simulink model "SSN_39busRT_Ctrl_4WT_19B"  (R2021a)
settings: Solver=ode3  StartTime=0.0  StopTime=10  FixedStep=Ts  MaxStep=1/60  RelTol=1e-2  AbsTol=1e-1
PreLoadFcn:
  | Ts=2.50e-6; ssn_ieee39_params; load('Pwf.mat');
InitFcn:
  | Ts=2.50e-6; ssn_ieee39_params; load('Pwf.mat');
values from neighbouring files (symbols this model uses):
  f = 50    [ssn_ieee39_params_ctrl.m]
  fNom = f    (= 60)    [ssn_ieee39_params_ctrl.m]
  ILR = 5.02    [ssn_ieee39_params_ctrl.m]
  IQMIN = 0.1    [ssn_ieee39_params_ctrl.m]
  ISCLIM = 1    [ssn_ieee39_params_ctrl.m]
  ITFpu = 1.10    (= 1.1)    [ssn_ieee39_params_ctrl.m]
  K = 1    [ssn_ieee39_params_ctrl.m]
  K1 = 1    [ssn_ieee39_params_ctrl.m]
  K2 = 2    [ssn_ieee39_params_ctrl.m]
  KCL = 1.04    [ssn_ieee39_params_ctrl.m]
  KFB = 0    [ssn_ieee39_params_ctrl.m]
  KFF = 1    [ssn_ieee39_params_ctrl.m]
  KFIX = 1    [ssn_ieee39_params_ctrl.m]
  KG = 1    [ssn_ieee39_params_ctrl.m]
  KIA = 59.91    [ssn_ieee39_params_ctrl.m]
  KIOEX = 0.0303    [ssn_ieee39_params_ctrl.m]
  KIUEX = 0.0303    [ssn_ieee39_params_ctrl.m]
  KIUOEX = 1    [ssn_ieee39_params_ctrl.m]
  KIUUEX = 1    [ssn_ieee39_params_ctrl.m]
  KLR = 22.47    [ssn_ieee39_params_ctrl.m]
  KM = 1    [ssn_ieee39_params_ctrl.m]
  KOEL = 0.24    [ssn_ieee39_params_ctrl.m]
  Kp = 1    [ssn_ieee39_params_ctrl.m]
  KPA = 30    [ssn_ieee39_params_ctrl.m]
  KPOEL = 1    [ssn_ieee39_params_ctrl.m]
  KPOEX = 0    [ssn_ieee39_params_ctrl.m]
  KPUEX = 0    [ssn_ieee39_params_ctrl.m]
  KSCALE = 0.319    [ssn_ieee39_params_ctrl.m]
  KUF = 0    [ssn_ieee39_params_ctrl.m]
  KUI = 0.001    [ssn_ieee39_params_ctrl.m]
  KUL = 0.24    [ssn_ieee39_params_ctrl.m]
  s = 10    [ssn_ieee39_params_ctrl.m]
  TA = 0.01    [ssn_ieee39_params_ctrl.m]
  Tadj = 0    [ssn_ieee39_params_ctrl.m]
  taps = [1 1 1.07 1.07 1.009 1.025 1 1.025 1.025 1.025]*1    [ssn_ieee39_params_ctrl.m]
  TF = 0.02    [ssn_ieee39_params_ctrl.m]
  TG = 0.024    [ssn_ieee39_params_ctrl.m]
  TINV = 0    [ssn_ieee39_params_ctrl.m]
  TIT = 0.1    [ssn_ieee39_params_ctrl.m]
  TL_10_11_len = 14    [ssn_ieee39_params_ctrl.m]
  TL_10_13_len = 14    [ssn_ieee39_params_ctrl.m]
  TL_13_14_len = 32    [ssn_ieee39_params_ctrl.m]
  TL_14_15_len = 70    [ssn_ieee39_params_ctrl.m]
  TL_15_16_len = 31.5    [ssn_ieee39_params_ctrl.m]
  TL_16_17_len = 26    [ssn_ieee39_params_ctrl.m]
  TL_16_19_len = 61    [ssn_ieee39_params_ctrl.m]
  TL_16_21_len = 46    [ssn_ieee39_params_ctrl.m]
  TL_16_24_len = 15    [ssn_ieee39_params_ctrl.m]
  TL_17_18_len = 26    [ssn_ieee39_params_ctrl.m]
  TL_17_27_len = 59    [ssn_ieee39_params_ctrl.m]
  TL_1_2_len = 134    [ssn_ieee39_params_ctrl.m]
  TL_1_39_len = 105    [ssn_ieee39_params_ctrl.m]
  TL_21_22_len = 47    [ssn_ieee39_params_ctrl.m]
  TL_22_23_len = 33    [ssn_ieee39_params_ctrl.m]
  TL_24_23_len = 88    [ssn_ieee39_params_ctrl.m]
  TL_25_26_len = 101    [ssn_ieee39_params_ctrl.m]
  TL_26_27_len = 46.5    [ssn_ieee39_params_ctrl.m]
  TL_26_28_len = 151    [ssn_ieee39_params_ctrl.m]
  TL_26_29_len = 200    [ssn_ieee39_params_ctrl.m]
  TL_28_29_len = 48    [ssn_ieee39_params_ctrl.m]
  TL_2_25_len = 28    [ssn_ieee39_params_ctrl.m]
  TL_2_2_len = 49    [ssn_ieee39_params_ctrl.m]
  TL_3_18_len = 42    [ssn_ieee39_params_ctrl.m]
  TL_3_4_len = 53    [ssn_ieee39_params_ctrl.m]
  TL_4_14_len = 33    [ssn_ieee39_params_ctrl.m]
  TL_4_5_len = 32.5    [ssn_ieee39_params_ctrl.m]
  TL_5_6_len = 14    [ssn_ieee39_params_ctrl.m]
  TL_5_8_len = 32    [ssn_ieee39_params_ctrl.m]
  TL_6_11_len = 26.5    [ssn_ieee39_params_ctrl.m]
  TL_6_7_len = 25.5    [ssn_ieee39_params_ctrl.m]
  TL_7_8_len = 15    [ssn_ieee39_params_ctrl.m]
  TL_8_9_len = 93    [ssn_ieee39_params_ctrl.m]
  TL_9_39_len = 136    [ssn_ieee39_params_ctrl.m]
  TOEL = 5.00    (= 5)    [ssn_ieee39_params_ctrl.m]
  TQREF = 0    [ssn_ieee39_params_ctrl.m]
  TQSCL = 0.012    [ssn_ieee39_params_ctrl.m]
  Ts_PMU = 1/1000    (= 0.001)    [ssn_ieee39_params_ctrl.m]
  TU1 = 0    [ssn_ieee39_params_ctrl.m]
  TU2 = 0    [ssn_ieee39_params_ctrl.m]
  TU3 = 0    [ssn_ieee39_params_ctrl.m]
  TU4 = 0    [ssn_ieee39_params_ctrl.m]
  TUL = 0    [ssn_ieee39_params_ctrl.m]
  TUP = 0.050    (= 0.05)    [ssn_ieee39_params_ctrl.m]
  TUQ = .005    (= 0.005)    [ssn_ieee39_params_ctrl.m]
  TUV = 0.2    [ssn_ieee39_params_ctrl.m]
  VAAMAX = VAMAX    (= 7.05)    [ssn_ieee39_params_ctrl.m]
  VAMAX = 7.05    [ssn_ieee39_params_ctrl.m]
  VAMIN = -6.11    [ssn_ieee39_params_ctrl.m]
  VBMAX = 999    [ssn_ieee39_params_ctrl.m]
  VF = 0    [ssn_ieee39_params_ctrl.m]
  VFB = 0    [ssn_ieee39_params_ctrl.m]
  VMMAX = 7.05    [ssn_ieee39_params_ctrl.m]
  VMMIN = -6.11    [ssn_ieee39_params_ctrl.m]
  VOELmax1 = 0.2353    [ssn_ieee39_params_ctrl.m]
  VOELmax2 = 0.0    (= 0)    [ssn_ieee39_params_ctrl.m]
  VOELmin1 = -0.24    [ssn_ieee39_params_ctrl.m]
  VOELmin2 = -1.0    (= -1)    [ssn_ieee39_params_ctrl.m]
  VRMAX = 7.05    [ssn_ieee39_params_ctrl.m]
  VRMIN = -6.11    [ssn_ieee39_params_ctrl.m]
  VSCLmax = 0.20    (= 0.2)    [ssn_ieee39_params_ctrl.m]
  VSCLmin = -0.10    (= -0.1)    [ssn_ieee39_params_ctrl.m]
  VUELmax1 = 1    [ssn_ieee39_params_ctrl.m]
  VUELmax2 = 1    [ssn_ieee39_params_ctrl.m]
  VUELmin1 = -1    [ssn_ieee39_params_ctrl.m]
  VUELmin2 = -1    [ssn_ieee39_params_ctrl.m]
  VUImax = 1    [ssn_ieee39_params_ctrl.m]
  VUImin = -1    [ssn_ieee39_params_ctrl.m]
undefined symbols (not defined in the file or in its folder): another_event_name, D1, Delta, DiscIntNeverNeededParam, find_system, MOV_segment9, my_event_name, powergui, Pw1, Pw2, Pw3, Pw4, vNomHV
libraries: powerlib_extras x162, spsThreePhaseVIMeasurementLib x55, spsCurrentMeasurementLib x52, simulink_extras x44, slpidlib x40, op_dpl_lib x36, spsST2AModel x20, spsThreePhaseParallelRLCLoadLib x20, spsThreePhaseTransformerTwoWindingsLib x17, spsControlledVoltageSourceLib x16, spsVoltageMeasurementLib x12, spsSynchronousMachinepuStandardLib x10
(part 6 of 19)

== system SSN_39busRT_Ctrl_4WT_19B/powergui/EquivalentModel16/Yout ==
  v,i : Inport
  Demux : Demux  Outputs=[1 1 1 1 1 1 1 1 1 1 1 1]
  tag scope: T56_4730_4741406695273=global, T56_4731_4743248439477=global, T56_4732_4745660404880=global, T72_6441_8594295325773=global, T72_6442_8596923134147=global, T72_6443_8599741842799=global, T80_6661_10245256504684=global, T80_6662_10243102637747=global, T80_6662_10245911720449=global, T80_6663_10243756033361=global, T80_6663_10246790665215=global, T80_6664_10244633157975=global
  wires:
  v,i/1 -> Demux/1
  Demux/1 -> [T72_6441_8594295325773]
  Demux/2 -> [T72_6442_8596923134147]
  Demux/3 -> [T72_6443_8599741842799]
  Demux/4 -> [T56_4730_4741406695273]
  Demux/5 -> [T56_4732_4745660404880]
  Demux/6 -> [T56_4731_4743248439477]
  Demux/7 -> [T80_6661_10245256504684]
  Demux/8 -> [T80_6662_10245911720449]
  Demux/9 -> [T80_6663_10246790665215]
  Demux/10 -> [T80_6662_10243102637747]
  Demux/11 -> [T80_6663_10243756033361]
  Demux/12 -> [T80_6664_10244633157975]

== system SSN_39busRT_Ctrl_4WT_19B/powergui/EquivalentModel17/Sources ==
  Mux : Mux  Inputs=[2 1 1 1 1 1 1 1 1 1]
  u : Outport  VectorParamsAs1DForOutWhenUnconnected=off
  wires:
  Mux/1 -> u/1
  [T65_5743_7340394662837] -> Mux/1
  [T76_6245_8362305392589] -> Mux/2
  [T76_6246_8363477414484] -> Mux/3
  [T76_6247_8364872173221] -> Mux/4
  [T75_6196_8146580275268] -> Mux/5
  [T75_6197_8147667563989] -> Mux/6
  [T75_6198_8148974225777] -> Mux/7
  [T75_6196_8148676870836] -> Mux/8
  [T75_6197_8149763564695] -> Mux/9
  [T75_6198_8151069631622] -> Mux/10

== system SSN_39busRT_Ctrl_4WT_19B/powergui/EquivalentModel17/Yout ==
  v,i : Inport
  Demux : Demux  Outputs=[2 1 1 1 1 1 1 1 1 1 1 1 1 1 1 1 1 1 1 1 1 1 1 1 1 1 1 1]
  tag scope: T55_4653_4627484077960=global, T55_4654_4629568952949=global, T55_4655_4631788251212=global, T56_4727_4745233583373=global, T56_4728_4743871655841=global, T56_4728_4747080717351=global, T56_4729_4742591329737=global, T56_4729_4745716943000=global, T56_4729_4749498425805=global, T56_4730_4741392605062=global, T56_4730_4744434770078=global, T56_4730_4748132683584=global, T56_4731_4739957074542=global, T56_4731_4743234198584=global, T56_4731_4746848542792=global, T56_4732_4741796921701=global, T56_4732_4745646003429=global, T56_4733_4744206865714=global, T65_5738_7276287426115=global, T78_6554_9761341477516=global, T78_6554_9763216670330=global, T78_6555_9761848914346=global, T78_6555_9763723549584=global, T78_6556_9762573376817=global, T78_6556_9764447454479=global, T79_6603_10014042814288=global, T79_6604_10014630189419=global, T79_6605_10015437941512=global
  wires:
  v,i/1 -> Demux/1
  Demux/1 -> [T65_5738_7276287426115]
  Demux/2 -> [T56_4727_4745233583373]
  Demux/3 -> [T56_4729_4749498425805]
  Demux/4 -> [T56_4728_4747080717351]
  Demux/5 -> [T56_4728_4743871655841]
  Demux/6 -> [T56_4730_4748132683584]
  Demux/7 -> [T56_4729_4745716943000]
  Demux/8 -> [T56_4729_4742591329737]
  Demux/9 -> [T56_4731_4746848542792]
  Demux/10 -> [T56_4730_4744434770078]
  Demux/11 -> [T56_4730_4741392605062]
  Demux/12 -> [T56_4732_4745646003429]
  Demux/13 -> [T56_4731_4743234198584]
  Demux/14 -> [T56_4731_4739957074542]
  Demux/15 -> [T56_4733_4744206865714]
  Demux/16 -> [T56_4732_4741796921701]
  Demux/17 -> [T79_6603_10014042814288]
  Demux/18 -> [T79_6604_10014630189419]
  Demux/19 -> [T79_6605_10015437941512]
  Demux/20 -> [T78_6554_9761341477516]
  Demux/21 -> [T78_6555_9761848914346]
  Demux/22 -> [T78_6556_9762573376817]
  Demux/23 -> [T78_6554_9763216670330]
  Demux/24 -> [T78_6555_9763723549584]
  Demux/25 -> [T78_6556_9764447454479]
  Demux/26 -> [T55_4653_4627484077960]
  Demux/27 -> [T55_4654_4629568952949]
  Demux/28 -> [T55_4655_4631788251212]

== system SSN_39busRT_Ctrl_4WT_19B/powergui/EquivalentModel18/Sources ==
  Mux : Mux  Inputs=[1 1 1 1 1 1]
  u : Outport  VectorParamsAs1DForOutWhenUnconnected=off
  wires:
  Mux/1 -> u/1
  [T76_6246_8359372382981] -> Mux/1
  [T76_6247_8360543323472] -> Mux/2
  [T76_6248_8361937000805] -> Mux/3
  [T76_6249_8355395478954] -> Mux/4
  [T76_6250_8356560405551] -> Mux/5
  [T76_6251_8357948068989] -> Mux/6

== system SSN_39busRT_Ctrl_4WT_19B/powergui/EquivalentModel18/Yout ==
  v,i : Inport
  Demux : Demux  Outputs=[1 1 1 1 1 1 1 1 1]
  tag scope: T56_4732_4739239959997=global, T56_4733_4741077859883=global, T56_4734_4743485728987=global, T79_6604_10010967878637=global, T79_6605_10011554239309=global, T79_6606_10012360976943=global, T79_6607_10005727568997=global, T79_6608_10006308288062=global, T79_6609_10007109384090=global
  wires:
  v,i/1 -> Demux/1
  Demux/1 -> [T56_4732_4739239959997]
  Demux/2 -> [T56_4734_4743485728987]
  Demux/3 -> [T56_4733_4741077859883]
  Demux/4 -> [T79_6604_10010967878637]
  Demux/5 -> [T79_6605_10011554239309]
  Demux/6 -> [T79_6606_10012360976943]
  Demux/7 -> [T79_6607_10005727568997]
  Demux/8 -> [T79_6608_10006308288062]
  Demux/9 -> [T79_6609_10007109384090]

== system SSN_39busRT_Ctrl_4WT_19B/powergui/EquivalentModel19/Sources ==
  Mux : Mux  Inputs=[1 1 1 1 1 1 1 1 1 1 1 1 1 1 1]
  u : Outport  VectorParamsAs1DForOutWhenUnconnected=off
  wires:
  Mux/1 -> u/1
  [T76_6248_8355999055039] -> Mux/1
  [T76_6249_8357166447881] -> Mux/2
  [T76_6250_8358556577565] -> Mux/3
  [T76_6250_8352783092665] -> Mux/4
  [T76_6251_8353946937858] -> Mux/5
  [T76_6252_8355333519893] -> Mux/6
  [T76_6252_8350236052370] -> Mux/7
  [T76_6253_8351396140089] -> Mux/8
  [T76_6254_8352778964651] -> Mux/9
  [T76_6245_8360654367305] -> Mux/10
  [T76_6246_8361827648147] -> Mux/11
  [T76_6247_8363223665832] -> Mux/12
  [T76_6248_8355359545726] -> Mux/13
  [T76_6249_8356527190358] -> Mux/14
  [T76_6250_8357917571832] -> Mux/15

== system SSN_39busRT_Ctrl_4WT_19B/powergui/EquivalentModel19/Yout ==
  v,i : Inport
  Demux : Demux  Outputs=[1 1 1 1 1 1 1 1 1 1 1 1 1 1 1 1 1 1]
  tag scope: T56_4733_4738286039607=global, T56_4734_4740122092675=global, T56_4735_4742527993909=global, T79_6603_10012751864210=global, T79_6604_10013340420354=global, T79_6605_10014149353460=global, T79_6606_10006333101250=global, T79_6606_10006888715093=global, T79_6607_10006916370091=global, T79_6607_10007471747731=global, T79_6608_10002961019338=global, T79_6608_10007720015894=global, T79_6608_10008275157332=global, T79_6609_10003540723944=global, T79_6610_10004340805511=global, T79_6610_9999627275735=global, T79_6611_10000203455472=global, T79_6612_10001000012171=global
  wires:
  v,i/1 -> Demux/1
  Demux/1 -> [T56_4733_4738286039607]
  Demux/2 -> [T56_4735_4742527993909]
  Demux/3 -> [T56_4734_4740122092675]
  Demux/4 -> [T79_6606_10006888715093]
  Demux/5 -> [T79_6607_10007471747731]
  Demux/6 -> [T79_6608_10008275157332]
  Demux/7 -> [T79_6608_10002961019338]
  Demux/8 -> [T79_6609_10003540723944]
  Demux/9 -> [T79_6610_10004340805511]
  Demux/10 -> [T79_6610_9999627275735]
  Demux/11 -> [T79_6611_10000203455472]
  Demux/12 -> [T79_6612_10001000012171]
  Demux/13 -> [T79_6603_10012751864210]
  Demux/14 -> [T79_6604_10013340420354]
  Demux/15 -> [T79_6605_10014149353460]
  Demux/16 -> [T79_6606_10006333101250]
  Demux/17 -> [T79_6607_10006916370091]
  Demux/18 -> [T79_6608_10007720015894]

== system SSN_39busRT_Ctrl_4WT_19B/powergui/EquivalentModel2/Sources ==
  Mux : Mux  Inputs=[1 1]
  u : Outport  VectorParamsAs1DForOutWhenUnconnected=off
  wires:
  Mux/1 -> u/1
  [T160_13858_40016383632279] -> Mux/1
  [T161_13907_39894470939587] -> Mux/2

== system SSN_39busRT_Ctrl_4WT_19B/powergui/EquivalentModel2/Yout ==
  v,i : Inport
  Demux : Demux  Outputs=[1 1 1]
  tag scope: T150_12991_36851941643877=global, T167_14636_46271938604014=global, T168_14685_46271433640443=global
  wires:
  v,i/1 -> Demux/1
  Demux/1 -> [T167_14636_46271938604014]
  Demux/2 -> [T168_14685_46271433640443]
  Demux/3 -> [T150_12991_36851941643877]

== system SSN_39busRT_Ctrl_4WT_19B/powergui/EquivalentModel20/Sources ==
  Mux : Mux  Inputs=[1 1 1 1 1 1]
  u : Outport  VectorParamsAs1DForOutWhenUnconnected=off
  wires:
  Mux/1 -> u/1
  [T76_6252_8349724495860] -> Mux/1
  [T76_6253_8350884793404] -> Mux/2
  [T76_6254_8352267827789] -> Mux/3
  [T75_6200_8142991377200] -> Mux/4
  [T75_6201_8144069994674] -> Mux/5
  [T75_6202_8145367985214] -> Mux/6

== system SSN_39busRT_Ctrl_4WT_19B/powergui/EquivalentModel20/Yout ==
  v,i : Inport
  Demux : Demux  Outputs=[1 1 1 1 1 1 1 1 1]
  tag scope: T56_4735_4736623003114=global, T56_4736_4738455362545=global, T56_4737_4740857328039=global, T78_6558_9755856196192=global, T78_6559_9756355505283=global, T78_6560_9757071840015=global, T79_6610_9999184791373=global, T79_6611_9999761167945=global, T79_6612_10000557921480=global
  wires:
  v,i/1 -> Demux/1
  Demux/1 -> [T56_4735_4736623003114]
  Demux/2 -> [T56_4737_4740857328039]
  Demux/3 -> [T56_4736_4738455362545]
  Demux/4 -> [T79_6610_9999184791373]
  Demux/5 -> [T79_6611_9999761167945]
  Demux/6 -> [T79_6612_10000557921480]
  Demux/7 -> [T78_6558_9755856196192]
  Demux/8 -> [T78_6559_9756355505283]
  Demux/9 -> [T78_6560_9757071840015]

== system SSN_39busRT_Ctrl_4WT_19B/powergui/EquivalentModel21/Sources ==
  Mux : Mux  Inputs=[2 2 1 1 1]
  u : Outport  VectorParamsAs1DForOutWhenUnconnected=off
  wires:
  Mux/1 -> u/1
  [T65_5745_7336353849760] -> Mux/1
  [T65_5747_7332463206010] -> Mux/2
  [T76_6253_8349626409858] -> Mux/3
  [T76_6254_8350784031332] -> Mux/4
  [T76_6255_8352164389647] -> Mux/5

== system SSN_39busRT_Ctrl_4WT_19B/powergui/EquivalentModel21/Yout ==
  v,i : Inport
  Demux : Demux  Outputs=[2 2 1 1 1 1 1 1 1 1 1 1 1 1 1 1 1 1 1 1 1 1 1]
  tag scope: T55_4651_4629921358801=global, T55_4652_4632010094694=global, T55_4653_4634233253859=global, T55_4655_4625292121246=global, T55_4656_4627373082108=global, T55_4657_4629588466242=global, T56_4728_4743880730792=global, T56_4729_4742517359948=global, T56_4729_4745726068179=global, T56_4730_4744360850516=global, T56_4730_4748141862282=global, T56_4731_4746774676750=global, T56_4733_4737635453373=global, T56_4734_4739471606896=global, T56_4735_4741877615169=global, T56_4736_4735913887010=global, T56_4737_4737744399623=global, T56_4738_4740144397247=global, T65_5740_7272266627846=global, T65_5742_7268395998904=global, T79_6611_9998460518046=global, T79_6612_9999034384210=global, T79_6613_9999828627335=global
  wires:
  v,i/1 -> Demux/1
  Demux/1 -> [T65_5740_7272266627846]
  Demux/2 -> [T65_5742_7268395998904]
  Demux/3 -> [T56_4736_4735913887010]
  Demux/4 -> [T56_4738_4740144397247]
  Demux/5 -> [T56_4737_4737744399623]
  Demux/6 -> [T56_4728_4743880730792]
  Demux/7 -> [T56_4730_4748141862282]
  Demux/8 -> [T56_4729_4745726068179]
  Demux/9 -> [T56_4729_4742517359948]
  Demux/10 -> [T56_4731_4746774676750]
  Demux/11 -> [T56_4730_4744360850516]
  Demux/12 -> [T56_4733_4737635453373]
  Demux/13 -> [T56_4735_4741877615169]
  Demux/14 -> [T56_4734_4739471606896]
  Demux/15 -> [T79_6611_9998460518046]
  Demux/16 -> [T79_6612_9999034384210]
  Demux/17 -> [T79_6613_9999828627335]
  Demux/18 -> [T55_4651_4629921358801]
  Demux/19 -> [T55_4652_4632010094694]
  Demux/20 -> [T55_4653_4634233253859]
  Demux/21 -> [T55_4655_4625292121246]
  Demux/22 -> [T55_4656_4627373082108]
  Demux/23 -> [T55_4657_4629588466242]

== system SSN_39busRT_Ctrl_4WT_19B/powergui/EquivalentModel22/Sources ==
  Mux : Mux  Inputs=[1 1 1 1 1 1 1 1 1]
  u : Outport  VectorParamsAs1DForOutWhenUnconnected=off
  wires:
  Mux/1 -> u/1
  [T76_6246_8360055680821] -> Mux/1
  [T76_6247_8361226495418] -> Mux/2
  [T76_6248_8362620046856] -> Mux/3
  [T76_6242_8366410502504] -> Mux/4
  [T76_6243_8367588622223] -> Mux/5
  [T76_6244_8368989478784] -> Mux/6
  [T75_6197_8144839329755] -> Mux/7
  [T75_6198_8145924716227] -> Mux/8
  [T75_6199_8147229475766] -> Mux/9

== system SSN_39busRT_Ctrl_4WT_19B/powergui/EquivalentModel22/Yout ==
  v,i : Inport
  Demux : Demux  Outputs=[1 1 1 1 1 1 1 1 1 1 1 1]
  tag scope: T56_4731_4740035422545=global, T56_4732_4741875219477=global, T56_4733_4744285109971=global, T78_6555_9759221588545=global, T78_6556_9759727242358=global, T78_6557_9760449921812=global, T79_6600_10019426700669=global, T79_6601_10020019796141=global, T79_6602_10020833268575=global, T79_6604_10011595241113=global, T79_6605_10012181483684=global, T79_6606_10012988103216=global
  wires:
  v,i/1 -> Demux/1
  Demux/1 -> [T56_4731_4740035422545]
  Demux/2 -> [T56_4733_4744285109971]
  Demux/3 -> [T56_4732_4741875219477]
  Demux/4 -> [T79_6604_10011595241113]
  Demux/5 -> [T79_6605_10012181483684]
  Demux/6 -> [T79_6606_10012988103216]
  Demux/7 -> [T79_6600_10019426700669]
  Demux/8 -> [T79_6601_10020019796141]
  Demux/9 -> [T79_6602_10020833268575]
  Demux/10 -> [T78_6555_9759221588545]
  Demux/11 -> [T78_6556_9759727242358]
  Demux/12 -> [T78_6557_9760449921812]

== system SSN_39busRT_Ctrl_4WT_19B/powergui/EquivalentModel23/Sources ==
  Mux : Mux  Inputs=[2 1 1 1 1 1 1]
  u : Outport  VectorParamsAs1DForOutWhenUnconnected=off
  wires:
  Mux/1 -> u/1
  [T65_5751_7325132426490] -> Mux/1
  [T76_6245_8361963326014] -> Mux/2
  [T76_6246_8363135431839] -> Mux/3
  [T76_6247_8364530274505] -> Mux/4
  [T76_6247_8357993829039] -> Mux/5
  [T76_6248_8359162597039] -> Mux/6
  [T76_6249_8360554101881] -> Mux/7

== system SSN_39busRT_Ctrl_4WT_19B/powergui/EquivalentModel23/Yout ==
  v,i : Inport
  Demux : Demux  Outputs=[2 1 1 1 1 1 1 1 1 1 1 1 1 1 1 1]
  tag scope: T55_4656_4624320770525=global, T55_4657_4626399774323=global, T55_4658_4628613201394=global, T56_4734_4736597044932=global, T56_4735_4735640237919=global, T56_4735_4738431351636=global, T56_4736_4737472697805=global, T56_4736_4740835392039=global, T56_4737_4739874770338=global, T65_5746_7261105249000=global, T79_6603_10013733675128=global, T79_6604_10014321128994=global, T79_6605_10009130640049=global, T79_6605_10015128959821=global, T79_6606_10009714962717=global, T79_6607_10010519662347=global
  wires:
  v,i/1 -> Demux/1
  Demux/1 -> [T65_5746_7261105249000]
  Demux/2 -> [T56_4734_4736597044932]
  Demux/3 -> [T56_4736_4740835392039]
  Demux/4 -> [T56_4735_4738431351636]
  Demux/5 -> [T56_4735_4735640237919]
  Demux/6 -> [T56_4737_4739874770338]
  Demux/7 -> [T56_4736_4737472697805]
  Demux/8 -> [T79_6603_10013733675128]
  Demux/9 -> [T79_6604_10014321128994]
  Demux/10 -> [T79_6605_10015128959821]
  Demux/11 -> [T79_6605_10009130640049]
  Demux/12 -> [T79_6606_10009714962717]
  Demux/13 -> [T79_6607_10010519662347]
  Demux/14 -> [T55_4656_4624320770525]
  Demux/15 -> [T55_4657_4626399774323]
  Demux/16 -> [T55_4658_4628613201394]

== system SSN_39busRT_Ctrl_4WT_19B/powergui/EquivalentModel24/Sources ==
  Mux : Mux  Inputs=[1 1 1 1 1 1]
  u : Outport  VectorParamsAs1DForOutWhenUnconnected=off
  wires:
  Mux/1 -> u/1
  [T76_6249_8354756178737] -> Mux/1
  [T76_6250_8355921357123] -> Mux/2
  [T76_6251_8357309272351] -> Mux/3
  [T76_6246_8358594215088] -> Mux/4
  [T76_6247_8359765449333] -> Mux/5
  [T76_6248_8361159420421] -> Mux/6

== system SSN_39busRT_Ctrl_4WT_19B/powergui/EquivalentModel24/Yout ==
  v,i : Inport
  Demux : Demux  Outputs=[1 1 1 1 1 1 1 1 1]
  tag scope: T56_4732_4738755463244=global, T56_4733_4740593463584=global, T56_4734_4743001439727=global, T79_6604_10010288835284=global, T79_6605_10010875471525=global, T79_6606_10011682484729=global, T79_6607_10005172148572=global, T79_6608_10005753103840=global, T79_6609_10006554436069=global
  wires:
  v,i/1 -> Demux/1
  Demux/1 -> [T56_4732_4738755463244]
  Demux/2 -> [T56_4734_4743001439727]
  Demux/3 -> [T56_4733_4740593463584]
  Demux/4 -> [T79_6607_10005172148572]
  Demux/5 -> [T79_6608_10005753103840]
  Demux/6 -> [T79_6609_10006554436069]
  Demux/7 -> [T79_6604_10010288835284]
  Demux/8 -> [T79_6605_10010875471525]
  Demux/9 -> [T79_6606_10011682484729]

== system SSN_39busRT_Ctrl_4WT_19B/powergui/EquivalentModel25/Sources ==
  Mux : Mux  Inputs=[2 1 1 1 1 1 1]
  u : Outport  VectorParamsAs1DForOutWhenUnconnected=off
  wires:
  Mux/1 -> u/1
  [T66_5785_7598354960298] -> Mux/1
  [T76_6250_8351956446770] -> Mux/2
  [T76_6251_8353120375893] -> Mux/3
  [T76_6252_8354507041858] -> Mux/4
  [T75_6196_8148127232584] -> Mux/5
  [T75_6197_8149213713993] -> Mux/6
  [T75_6198_8150519568468] -> Mux/7

== system SSN_39busRT_Ctrl_4WT_19B/powergui/EquivalentModel25/Yout ==
  v,i : Inport
  Demux : Demux  Outputs=[2 1 1 1 1 1 1 1 1 1 1 1 1 1 1 1]
  tag scope: T55_4658_4622627324357=global, T55_4659_4624702414027=global, T55_4660_4626911926970=global, T56_4733_4737879890857=global, T56_4734_4739715994153=global, T56_4735_4742121948906=global, T56_4736_4734765032334=global, T56_4737_4736595645403=global, T56_4738_4738995750065=global, T66_5780_7532793078147=global, T78_6554_9762638548620=global, T78_6555_9763145228740=global, T78_6556_9763868934501=global, T79_6608_10002185930088=global, T79_6609_10002765713427=global, T79_6610_10003565873729=global
  wires:
  v,i/1 -> Demux/1
  Demux/1 -> [T66_5780_7532793078147]
  Demux/2 -> [T56_4733_4737879890857]
  Demux/3 -> [T56_4735_4742121948906]
  Demux/4 -> [T56_4734_4739715994153]
  Demux/5 -> [T56_4736_4734765032334]
  Demux/6 -> [T56_4738_4738995750065]
  Demux/7 -> [T56_4737_4736595645403]
  Demux/8 -> [T79_6608_10002185930088]
  Demux/9 -> [T79_6609_10002765713427]
  Demux/10 -> [T79_6610_10003565873729]
  Demux/11 -> [T78_6554_9762638548620]
  Demux/12 -> [T78_6555_9763145228740]
  Demux/13 -> [T78_6556_9763868934501]
  Demux/14 -> [T55_4658_4622627324357]
  Demux/15 -> [T55_4659_4624702414027]
  Demux/16 -> [T55_4660_4626911926970]

== system SSN_39busRT_Ctrl_4WT_19B/powergui/EquivalentModel26/Sources ==
  Mux : Mux  Inputs=[1 1 1 1 1 1 1 1 1 1 1 1]
  u : Outport  VectorParamsAs1DForOutWhenUnconnected=off
  wires:
  Mux/1 -> u/1
  [T76_6251_8351349994293] -> Mux/1
  [T76_6252_8352511457170] -> Mux/2
  [T76_6253_8353895656889] -> Mux/3
  [T77_6297_8571747053055] -> Mux/4
  [T77_6298_8573000936818] -> Mux/5
  [T77_6299_8574480921620] -> Mux/6
  [T76_6253_8347416066484] -> Mux/7
  [T76_6254_8348574569221] -> Mux/8
  [T76_6255_8349955808800] -> Mux/9
  [T76_6254_8346184924105] -> Mux/10
  [T76_6255_8347341548105] -> Mux/11
  [T76_6256_8348720908947] -> Mux/12

== system SSN_39busRT_Ctrl_4WT_19B/powergui/EquivalentModel26/Yout ==
  v,i : Inport
  Demux : Demux  Outputs=[1 1 1 1 1 1 1 1 1 1 1 1 1 1 1 1 1 1 1 1 1]
  tag scope: T56_4734_4736924527156=global, T56_4735_4738758783633=global, T56_4736_4741162770516=global, T79_6609_10001022123259=global, T79_6610_10001599593025=global, T79_6611_10002397439753=global, T79_6611_9996542631766=global, T79_6612_9994916609526=global, T79_6612_9997117324638=global, T79_6613_9995489539964=global, T79_6613_9997912394473=global, T79_6614_9996282847364=global, T80_6655_10260165963797=global, T80_6656_10260830699437=global, T80_6657_10261719164076=global, T81_7051_10262087113735=global, T81_7052_10265770741383=global, T81_7053_10269675335944=global, T81_7063_10334482697438=global, T81_7064_10338134091012=global, T81_7065_10342006451500=global
  wires:
  v,i/1 -> Demux/1
  Demux/1 -> [T56_4734_4736924527156]
  Demux/2 -> [T56_4736_4741162770516]
  Demux/3 -> [T56_4735_4738758783633]
  Demux/4 -> [T79_6609_10001022123259]
  Demux/5 -> [T79_6610_10001599593025]
  Demux/6 -> [T79_6611_10002397439753]
  Demux/7 -> [T80_6655_10260165963797]
  Demux/8 -> [T80_6656_10260830699437]
  Demux/9 -> [T80_6657_10261719164076]
  Demux/10 -> [T79_6611_9996542631766]
  Demux/11 -> [T79_6612_9997117324638]
  Demux/12 -> [T79_6613_9997912394473]
  Demux/13 -> [T79_6612_9994916609526]
  Demux/14 -> [T79_6613_9995489539964]
  Demux/15 -> [T79_6614_9996282847364]
  Demux/16 -> [T81_7063_10334482697438]
  Demux/17 -> [T81_7064_10338134091012]
  Demux/18 -> [T81_7065_10342006451500]
  Demux/19 -> [T81_7051_10262087113735]
  Demux/20 -> [T81_7052_10265770741383]
  Demux/21 -> [T81_7053_10269675335944]

== system SSN_39busRT_Ctrl_4WT_19B/powergui/EquivalentModel27/Sources ==
  Mux : Mux  Inputs=[1 1 1 1 1 1]
  u : Outport  VectorParamsAs1DForOutWhenUnconnected=off
  wires:
  Mux/1 -> u/1
  [T76_6252_8349126481072] -> Mux/1
  [T76_6253_8350286820581] -> Mux/2
  [T76_6254_8351669896932] -> Mux/3
  [T77_6298_8571212545567] -> Mux/4
  [T77_6299_8572463951746] -> Mux/5
  [T77_6300_8573941458964] -> Mux/6

== system SSN_39busRT_Ctrl_4WT_19B/powergui/EquivalentModel27/Yout ==
  v,i : Inport
  Demux : Demux  Outputs=[1 1 1 1 1 1 1 1 1]
  tag scope: T56_4735_4736050764883=global, T56_4736_4737883174542=global, T56_4737_4740285193555=global, T79_6610_9998619656599=global, T79_6611_9999196072538=global, T79_6612_9999992865440=global, T80_6656_10259066586252=global, T80_6657_10259728995809=global, T80_6658_10260615134366=global
  wires:
  v,i/1 -> Demux/1
  Demux/1 -> [T56_4735_4736050764883]
  Demux/2 -> [T56_4737_4740285193555]
  Demux/3 -> [T56_4736_4737883174542]
  Demux/4 -> [T79_6610_9998619656599]
  Demux/5 -> [T79_6611_9999196072538]
  Demux/6 -> [T79_6612_9999992865440]
  Demux/7 -> [T80_6656_10259066586252]
  Demux/8 -> [T80_6657_10259728995809]
  Demux/9 -> [T80_6658_10260615134366]

== system SSN_39busRT_Ctrl_4WT_19B/powergui/EquivalentModel28/Sources ==
  Mux : Mux  Inputs=[1 1 1 1 1 1]
  u : Outport  VectorParamsAs1DForOutWhenUnconnected=off
  wires:
  Mux/1 -> u/1
  [T76_6254_8346805107747] -> Mux/1
  [T76_6255_8347961144239] -> Mux/2
  [T76_6256_8349339917572] -> Mux/3
  [T76_6256_8342768243439] -> Mux/4
  [T76_6257_8343921529614] -> Mux/5
  [T76_6258_8345297552632] -> Mux/6

== system SSN_39busRT_Ctrl_4WT_19B/powergui/EquivalentModel28/Yout ==
  v,i : Inport
  Demux : Demux  Outputs=[1 1 1 1 1 1 1 1 1]
  tag scope: T56_4736_4735258604039=global, T56_4737_4737089166880=global, T56_4738_4739489218023=global, T79_6612_9995374656537=global, T79_6613_9995947035836=global, T79_6614_9990845763944=global, T79_6614_9996739792097=global, T79_6615_9991415563184=global, T79_6616_9992205739387=global
  wires:
  v,i/1 -> Demux/1
  Demux/1 -> [T56_4736_4735258604039]
  Demux/2 -> [T56_4738_4739489218023]
  Demux/3 -> [T56_4737_4737089166880]
  Demux/4 -> [T79_6612_9995374656537]
  Demux/5 -> [T79_6613_9995947035836]
  Demux/6 -> [T79_6614_9996739792097]
  Demux/7 -> [T79_6614_9990845763944]
  Demux/8 -> [T79_6615_9991415563184]
  Demux/9 -> [T79_6616_9992205739387]

== system SSN_39busRT_Ctrl_4WT_19B/powergui/EquivalentModel29/Sources ==
  Mux : Mux  Inputs=[1 1 1 1 1 1 1 1 1]
  u : Outport  VectorParamsAs1DForOutWhenUnconnected=off
  wires:
  Mux/1 -> u/1
  [T77_6303_8557517344221] -> Mux/1
  [T77_6304_8558761626948] -> Mux/2
  [T77_6305_8560232010714] -> Mux/3
  [T76_6255_8345572405200] -> Mux/4
  [T76_6256_8346726562954] -> Mux/5
  [T76_6257_8348103457551] -> Mux/6
  [T76_6257_8342152952688] -> Mux/7
  [T76_6258_8343303772618] -> Mux/8
  [T76_6259_8344677329389] -> Mux/9

== system SSN_39busRT_Ctrl_4WT_19B/powergui/EquivalentModel29/Yout ==
  v,i : Inport
  Demux : Demux  Outputs=[1 1 1 1 1 1 1 1 1 1 1 1]
  tag scope: T56_4737_4734548044623=global, T56_4738_4736376760646=global, T56_4739_4738774843919=global, T79_6613_9993747191104=global, T79_6614_9994317807968=global, T79_6615_9989673781496=global, T79_6615_9995108801795=global, T79_6616_9990241267163=global, T79_6617_9991029129792=global, T80_6661_10244209418922=global, T80_6662_10244865140619=global, T80_6663_10245744591315=global
  wires:
  v,i/1 -> Demux/1
  Demux/1 -> [T56_4737_4734548044623]
  Demux/2 -> [T56_4739_4738774843919]
  Demux/3 -> [T56_4738_4736376760646]
  Demux/4 -> [T80_6661_10244209418922]
  Demux/5 -> [T80_6662_10244865140619]
  Demux/6 -> [T80_6663_10245744591315]
  Demux/7 -> [T79_6613_9993747191104]
  Demux/8 -> [T79_6614_9994317807968]
  Demux/9 -> [T79_6615_9995108801795]
  Demux/10 -> [T79_6615_9989673781496]
  Demux/11 -> [T79_6616_9990241267163]
  Demux/12 -> [T79_6617_9991029129792]

== system SSN_39busRT_Ctrl_4WT_19B/powergui/EquivalentModel3/Sources ==
  Mux : Mux  Inputs=[1 1]
  u : Outport  VectorParamsAs1DForOutWhenUnconnected=off
  wires:
  Mux/1 -> u/1
  [T159_13813_39425934886620] -> Mux/1
  [T160_13862_39305619355219] -> Mux/2

== system SSN_39busRT_Ctrl_4WT_19B/powergui/EquivalentModel3/Yout ==
  v,i : Inport
  Demux : Demux  Outputs=[1 1 1]
  tag scope: T149_12946_36305397553553=global, T166_14591_45616211582443=global, T167_14640_45617278812063=global
  wires:
  v,i/1 -> Demux/1
  Demux/1 -> [T166_14591_45616211582443]
  Demux/2 -> [T167_14640_45617278812063]
  Demux/3 -> [T149_12946_36305397553553]

== system SSN_39busRT_Ctrl_4WT_19B/powergui/EquivalentModel30/Sources ==
  Mux : Mux  Inputs=[1 1 1 1 1 1 1 1 1]
  u : Outport  VectorParamsAs1DForOutWhenUnconnected=off
  wires:
  Mux/1 -> u/1
  [T74_6145_7942558741431] -> Mux/1
  [T74_6146_7943561365244] -> Mux/2
  [T74_6147_7944779998787] -> Mux/3
  [T75_6199_8143663390944] -> Mux/4
  [T75_6200_8144744463038] -> Mux/5
  [T75_6201_8146044908198] -> Mux/6
  [T74_6146_7939506225030] -> Mux/7
  [T74_6147_7940507783060] -> Mux/8
  [T74_6148_7941725350820] -> Mux/9

== system SSN_39busRT_Ctrl_4WT_19B/powergui/EquivalentModel30/Yout ==
  v,i : Inport
  Demux : Demux  Outputs=[1 1 1 1 1 1 1 1 1 1 1 1 1 1 1]
  tag scope: T54_4603_4508361632453=global, T54_4604_4510303875028=global, T54_4605_4512377237973=global, T55_4681_4616064652916=global, T55_4682_4617764664323=global, T55_4683_4620030048552=global, T77_6503_9520048468920=global, T77_6504_9516866878920=global, T77_6504_9520476153828=global, T77_6505_9517293565694=global, T77_6505_9521117513800=global, T77_6506_9517933927532=global, T78_6557_9757078334279=global, T78_6558_9757579944136=global, T78_6559_9758298579634=global
  wires:
  v,i/1 -> Demux/1
  Demux/1 -> [T55_4681_4616064652916]
  Demux/2 -> [T55_4683_4620030048552]
  Demux/3 -> [T55_4682_4617764664323]
  Demux/4 -> [T77_6503_9520048468920]
  Demux/5 -> [T77_6504_9520476153828]
  Demux/6 -> [T77_6505_9521117513800]
  Demux/7 -> [T78_6557_9757078334279]
  Demux/8 -> [T78_6558_9757579944136]
  Demux/9 -> [T78_6559_9758298579634]
  Demux/10 -> [T77_6504_9516866878920]
  Demux/11 -> [T77_6505_9517293565694]
  Demux/12 -> [T77_6506_9517933927532]
  Demux/13 -> [T54_4603_4508361632453]
  Demux/14 -> [T54_4604_4510303875028]
  Demux/15 -> [T54_4605_4512377237973]

== system SSN_39busRT_Ctrl_4WT_19B/powergui/EquivalentModel31/Sources ==
  Mux : Mux  Inputs=[2 1 1 1 1 1 1 1 1 1 1 1 1]
  u : Outport  VectorParamsAs1DForOutWhenUnconnected=off
  wires:
  Mux/1 -> u/1
  [T65_5741_7344585645240] -> Mux/1
  [T74_6149_7935135192316] -> Mux/2
  [T74_6150_7936130799173] -> Mux/3
  [T74_6151_7937342415759] -> Mux/4
  [T74_6152_7929459751575] -> Mux/5
  [T74_6153_7930450612057] -> Mux/6
  [T74_6154_7931657482268] -> Mux/7
  [T75_6195_8149342197297] -> Mux/8
  [T75_6196_8150431345777] -> Mux/9
  [T75_6197_8151739867323] -> Mux/10
  [T74_6152_7929055167392] -> Mux/11
  [T74_6153_7930046199987] -> Mux/12
  [T74_6154_7931253242312] -> Mux/13

== system SSN_39busRT_Ctrl_4WT_19B/powergui/EquivalentModel31/Yout ==
  v,i : Inport
  Demux : Demux  Outputs=[2 1 1 1 1 1 1 1 1 1 1 1 1 1 1 1 1 1 1 1 1 1 1 1 1]
  tag scope: T55_4652_4628704683953=global, T55_4653_4630791516007=global, T55_4654_4633012771333=global, T55_4683_4613781756552=global, T55_4684_4612758249279=global, T55_4684_4615478123111=global, T55_4685_4614452793414=global, T55_4685_4617739618249=global, T55_4686_4616712344007=global, T56_4730_4741240287269=global, T56_4731_4743081981247=global, T56_4732_4745493893130=global, T65_5736_7280458393712=global, T77_6507_9511275102386=global, T77_6508_9511696215728=global, T77_6509_9512331004135=global, T77_6510_9504364460041=global, T77_6510_9504712795202=global, T77_6511_9504781289467=global, T77_6511_9505129463438=global, T77_6512_9505411793958=global, T77_6512_9505759806740=global, T78_6553_9764432628859=global, T78_6554_9764941808879=global, T78_6555_9765668014540=global
  wires:
  v,i/1 -> Demux/1
  Demux/1 -> [T65_5736_7280458393712]
  Demux/2 -> [T56_4730_4741240287269]
  Demux/3 -> [T56_4732_4745493893130]
  Demux/4 -> [T56_4731_4743081981247]
  Demux/5 -> [T55_4683_4613781756552]
  Demux/6 -> [T55_4685_4617739618249]
  Demux/7 -> [T55_4684_4615478123111]
  Demux/8 -> [T55_4684_4612758249279]
  Demux/9 -> [T55_4686_4616712344007]
  Demux/10 -> [T55_4685_4614452793414]
  Demux/11 -> [T77_6507_9511275102386]
  Demux/12 -> [T77_6508_9511696215728]
  Demux/13 -> [T77_6509_9512331004135]
  Demux/14 -> [T77_6510_9504712795202]
  Demux/15 -> [T77_6511_9505129463438]
  Demux/16 -> [T77_6512_9505759806740]
  Demux/17 -> [T78_6553_9764432628859]
  Demux/18 -> [T78_6554_9764941808879]
  Demux/19 -> [T78_6555_9765668014540]
  Demux/20 -> [T77_6510_9504364460041]
  Demux/21 -> [T77_6511_9504781289467]
  Demux/22 -> [T77_6512_9505411793958]
  Demux/23 -> [T55_4652_4628704683953]
  Demux/24 -> [T55_4653_4630791516007]
  Demux/25 -> [T55_4654_4633012771333]

== system SSN_39busRT_Ctrl_4WT_19B/powergui/EquivalentModel32/Sources ==
  Mux : Mux  Inputs=[2 1 1 1 1 1 1]
  u : Outport  VectorParamsAs1DForOutWhenUnconnected=off
  wires:
  Mux/1 -> u/1
  [T65_5739_7348926796971] -> Mux/1
  [T75_6201_8142059340631] -> Mux/2
  [T75_6202_8143135758425] -> Mux/3
  [T75_6203_8144431549286] -> Mux/4
  [T75_6208_8127690328584] -> Mux/5
  [T75_6209_8128756022533] -> Mux/6
  [T75_6210_8130041089550] -> Mux/7

== system SSN_39busRT_Ctrl_4WT_19B/powergui/EquivalentModel32/Yout ==
  v,i : Inport
  Demux : Demux  Outputs=[2 1 1 1 1 1 1 1 1 1 1 1 1 1 1 1]
  tag scope: T55_4654_4626513286397=global, T55_4655_4628596151098=global, T55_4656_4630813439071=global, T56_4732_4738916855987=global, T56_4733_4740754806101=global, T56_4734_4743162728724=global, T56_4738_4733259425451=global, T56_4739_4735086344883=global, T56_4740_4737482513805=global, T65_5734_7284779530635=global, T78_6559_9754444085954=global, T78_6560_9754941333240=global, T78_6561_9755655606167=global, T78_6566_9738118288080=global, T78_6567_9738605483685=global, T78_6568_9739309704930=global
  wires:
  v,i/1 -> Demux/1
  Demux/1 -> [T65_5734_7284779530635]
  Demux/2 -> [T56_4732_4738916855987]
  Demux/3 -> [T56_4734_4743162728724]
  Demux/4 -> [T56_4733_4740754806101]
  Demux/5 -> [T56_4738_4733259425451]
  Demux/6 -> [T56_4740_4737482513805]
  Demux/7 -> [T56_4739_4735086344883]
  Demux/8 -> [T78_6559_9754444085954]
  Demux/9 -> [T78_6560_9754941333240]
  Demux/10 -> [T78_6561_9755655606167]
  Demux/11 -> [T78_6566_9738118288080]
  Demux/12 -> [T78_6567_9738605483685]
  Demux/13 -> [T78_6568_9739309704930]
  Demux/14 -> [T55_4654_4626513286397]
  Demux/15 -> [T55_4655_4628596151098]
  Demux/16 -> [T55_4656_4630813439071]

== system SSN_39busRT_Ctrl_4WT_19B/powergui/EquivalentModel33/Sources ==
  Mux : Mux  Inputs=[1 1 1 1 1 1 1 1 1]
  u : Outport  VectorParamsAs1DForOutWhenUnconnected=off
  wires:
  Mux/1 -> u/1
  [T74_6147_7938771902734] -> Mux/1
  [T74_6148_7939771018069] -> Mux/2
  [T74_6149_7940986143134] -> Mux/3
  [T75_6196_8147679523124] -> Mux/4
  [T75_6197_8148766386944] -> Mux/5
  [T75_6198_8150072623831] -> Mux/6
  [T74_6148_7935872410872] -> Mux/7
  [T74_6149_7936870460424] -> Mux/8
  [T74_6150_7938084519706] -> Mux/9

== system SSN_39busRT_Ctrl_4WT_19B/powergui/EquivalentModel33/Yout ==
  v,i : Inport
  Demux : Demux  Outputs=[1 1 1 1 1 1 1 1 1 1 1 1 1 1 1]
  tag scope: T54_4604_4507243268459=global, T54_4605_4509183577596=global, T54_4606_4511255007103=global, T55_4682_4614883891098=global, T55_4683_4616582080081=global, T55_4684_4618845519764=global, T77_6505_9515589606733=global, T77_6506_9512555048120=global, T77_6506_9516014005858=global, T77_6507_9512978449111=global, T77_6507_9516652080048=global, T77_6508_9513615525167=global, T78_6554_9762298099074=global, T78_6555_9762805137636=global, T78_6556_9763529201838=global
  wires:
  v,i/1 -> Demux/1
  Demux/1 -> [T55_4682_4614883891098]
  Demux/2 -> [T55_4684_4618845519764]
  Demux/3 -> [T55_4683_4616582080081]
  Demux/4 -> [T77_6505_9515589606733]
  Demux/5 -> [T77_6506_9516014005858]
  Demux/6 -> [T77_6507_9516652080048]
  Demux/7 -> [T78_6554_9762298099074]
  Demux/8 -> [T78_6555_9762805137636]
  Demux/9 -> [T78_6556_9763529201838]
  Demux/10 -> [T77_6506_9512555048120]
  Demux/11 -> [T77_6507_9512978449111]
  Demux/12 -> [T77_6508_9513615525167]
  Demux/13 -> [T54_4604_4507243268459]
  Demux/14 -> [T54_4605_4509183577596]
  Demux/15 -> [T54_4606_4511255007103]

== system SSN_39busRT_Ctrl_4WT_19B/powergui/EquivalentModel34/Sources ==
  Mux : Mux  Inputs=[1 1 1 1 1 1 1 1 1 1 1 1]
  u : Outport  VectorParamsAs1DForOutWhenUnconnected=off
  wires:
  Mux/1 -> u/1
  [T75_6196_8147746255903] -> Mux/1
  [T75_6197_8148832992252] -> Mux/2
  [T75_6198_8150139101668] -> Mux/3
  [T74_6153_7928716598417] -> Mux/4
  [T74_6154_7929705016203] -> Mux/5
  [T74_6155_7930909443719] -> Mux/6
  [T74_6153_7928312156314] -> Mux/7
  [T74_6154_7929300746214] -> Mux/8
  [T74_6155_7930505345844] -> Mux/9
  [T74_6157_7922089633427] -> Mux/10
  [T74_6158_7923071206370] -> Mux/11
  [T74_6159_7924268789043] -> Mux/12

== system SSN_39busRT_Ctrl_4WT_19B/powergui/EquivalentModel34/Yout ==
  v,i : Inport
  Demux : Demux  Outputs=[1 1 1 1 1 1 1 1 1 1 1 1 1 1 1 1 1 1]
  tag scope: T55_4685_4611813369279=global, T55_4686_4610947116552=global, T55_4686_4613506090990=global, T55_4687_4612638015838=global, T55_4687_4615763697037=global, T55_4688_4614893677340=global, T77_6511_9503079167211=global, T77_6511_9503427371217=global, T77_6512_9503493708988=global, T77_6512_9503841751805=global, T77_6513_9504121925830=global, T77_6513_9504469807457=global, T77_6515_9495460663397=global, T77_6516_9495868633609=global, T77_6517_9496490278886=global, T78_6554_9762332292776=global, T78_6555_9762839211856=global, T78_6556_9763563156578=global
  wires:
  v,i/1 -> Demux/1
  Demux/1 -> [T55_4685_4611813369279]
  Demux/2 -> [T55_4687_4615763697037]
  Demux/3 -> [T55_4686_4613506090990]
  Demux/4 -> [T55_4686_4610947116552]
  Demux/5 -> [T55_4688_4614893677340]
  Demux/6 -> [T55_4687_4612638015838]
  Demux/7 -> [T78_6554_9762332292776]
  Demux/8 -> [T78_6555_9762839211856]
  Demux/9 -> [T78_6556_9763563156578]
  Demux/10 -> [T77_6511_9503427371217]
  Demux/11 -> [T77_6512_9503841751805]
  Demux/12 -> [T77_6513_9504469807457]
  Demux/13 -> [T77_6511_9503079167211]
  Demux/14 -> [T77_6512_9503493708988]
  Demux/15 -> [T77_6513_9504121925830]
  Demux/16 -> [T77_6515_9495460663397]
  Demux/17 -> [T77_6516_9495868633609]
  Demux/18 -> [T77_6517_9496490278886]

== system SSN_39busRT_Ctrl_4WT_19B/powergui/EquivalentModel4/Sources ==
  Mux : Mux  Inputs=[1 1]
  u : Outport  VectorParamsAs1DForOutWhenUnconnected=off
  wires:
  Mux/1 -> u/1
  [T160_13863_39991555111447] -> Mux/1
  [T161_13912_39869752064095] -> Mux/2

== system SSN_39busRT_Ctrl_4WT_19B/powergui/EquivalentModel4/Yout ==
  v,i : Inport
  Demux : Demux  Outputs=[1 1 1]
  tag scope: T150_12996_36828272907374=global, T167_14641_46245399536655=global, T168_14690_46245000738081=global
  wires:
  v,i/1 -> Demux/1
  Demux/1 -> [T167_14641_46245399536655]
  Demux/2 -> [T168_14690_46245000738081]
  Demux/3 -> [T150_12996_36828272907374]

== system SSN_39busRT_Ctrl_4WT_19B/powergui/EquivalentModel5/Sources ==
  Mux : Mux  Inputs=[1 1 1 1 1 1 1 1 1]
  u : Outport  VectorParamsAs1DForOutWhenUnconnected=off
  wires:
  Mux/1 -> u/1
  [T76_6251_8352176570489] -> Mux/1
  [T76_6252_8353337949437] -> Mux/2
  [T76_6253_8354722065226] -> Mux/3
  [T76_6253_8349115027593] -> Mux/4
  [T76_6254_8350272858891] -> Mux/5
  [T76_6255_8351653427032] -> Mux/6
  [T76_6253_8348517047654] -> Mux/7
  [T76_6254_8349674920918] -> Mux/8
  [T76_6255_8351055531023] -> Mux/9

== system SSN_39busRT_Ctrl_4WT_19B/powergui/EquivalentModel5/Yout ==
  v,i : Inport
  Demux : Demux  Outputs=[1 1 1 1 1 1 1 1 1 1 1 1]
  tag scope: T56_4734_4737413720646=global, T56_4735_4739247926896=global, T56_4736_4741651860260=global, T79_6609_10001797148036=global, T79_6610_10002374539068=global, T79_6611_10003172307063=global, T79_6611_9997453092327=global, T79_6611_9998018194865=global, T79_6612_9998027194693=global, T79_6612_9998592257864=global, T79_6613_9998821674021=global, T79_6613_9999386697825=global
  wires:
  v,i/1 -> Demux/1
  Demux/1 -> [T56_4734_4737413720646]
  Demux/2 -> [T56_4736_4741651860260]
  Demux/3 -> [T56_4735_4739247926896]
  Demux/4 -> [T79_6609_10001797148036]
  Demux/5 -> [T79_6610_10002374539068]
  Demux/6 -> [T79_6611_10003172307063]
  Demux/7 -> [T79_6611_9998018194865]
  Demux/8 -> [T79_6612_9998592257864]
  Demux/9 -> [T79_6613_9999386697825]
  Demux/10 -> [T79_6611_9997453092327]
  Demux/11 -> [T79_6612_9998027194693]
  Demux/12 -> [T79_6613_9998821674021]

== system SSN_39busRT_Ctrl_4WT_19B/powergui/EquivalentModel6/Sources ==
  Mux : Mux  Inputs=[1 1 1 1 1 1]
  u : Outport  VectorParamsAs1DForOutWhenUnconnected=off
  wires:
  Mux/1 -> u/1
  [T74_6143_7946495708406] -> Mux/1
  [T74_6144_7947501840698] -> Mux/2
  [T74_6145_7948723982719] -> Mux/3
  [T75_6200_8142733175719] -> Mux/4
  [T75_6201_8143812048133] -> Mux/5
  [T75_6202_8145110293614] -> Mux/6

== system SSN_39busRT_Ctrl_4WT_19B/powergui/EquivalentModel6/Yout ==
  v,i : Inport
  Demux : Demux  Outputs=[1 1 1 1 1 1 1 1 1]
  tag scope: T55_4679_4618662058370=global, T55_4680_4620365714626=global, T55_4681_4622634987946=global, T77_6501_9524651688947=global, T77_6502_9525082659638=global, T77_6503_9525727305393=global, T78_6558_9755667907101=global, T78_6559_9756167455153=global, T78_6560_9756884028846=global
  wires:
  v,i/1 -> Demux/1
  Demux/1 -> [T55_4679_4618662058370]
  Demux/2 -> [T55_4681_4622634987946]
  Demux/3 -> [T55_4680_4620365714626]
  Demux/4 -> [T77_6501_9524651688947]
  Demux/5 -> [T77_6502_9525082659638]
  Demux/6 -> [T77_6503_9525727305393]
  Demux/7 -> [T78_6558_9755667907101]
  Demux/8 -> [T78_6559_9756167455153]
  Demux/9 -> [T78_6560_9756884028846]

== system SSN_39busRT_Ctrl_4WT_19B/powergui/EquivalentModel7/Sources ==
  Mux : Mux  Inputs=[2 1 1 1 1 1 1]
  u : Outport  VectorParamsAs1DForOutWhenUnconnected=off
  wires:
  Mux/1 -> u/1
  [T65_5749_7328722731587] -> Mux/1
  [T76_6243_8365815834391] -> Mux/2
  [T76_6244_8366991487865] -> Mux/3
  [T76_6245_8368389878181] -> Mux/4
  [T76_6244_8362560940218] -> Mux/5
  [T76_6245_8363735512288] -> Mux/6
  [T76_6246_8365132821200] -> Mux/7

== system SSN_39busRT_Ctrl_4WT_19B/powergui/EquivalentModel7/Yout ==
  v,i : Inport
  Demux : Demux  Outputs=[2 1 1 1 1 1 1 1 1 1 1 1 1 1 1 1]
  tag scope: T56_4702_4750302846636=global, T56_4703_4752532395919=global, T56_4704_4754899674130=global, T56_4730_4741235590532=global, T56_4731_4743077234282=global, T56_4732_4745489092646=global, T57_4780_4867595741341=global, T57_4781_4869577586341=global, T57_4782_4872134054868=global, T65_5744_7264675539288=global, T79_6601_10018273794664=global, T79_6602_10014889306339=global, T79_6602_10018864576563=global, T79_6603_10015479073778=global, T79_6603_10019675735424=global, T79_6604_10016289218179=global
  wires:
  v,i/1 -> Demux/1
  Demux/1 -> [T65_5744_7264675539288]
  Demux/2 -> [T56_4730_4741235590532]
  Demux/3 -> [T56_4732_4745489092646]
  Demux/4 -> [T56_4731_4743077234282]
  Demux/5 -> [T57_4780_4867595741341]
  Demux/6 -> [T57_4782_4872134054868]
  Demux/7 -> [T57_4781_4869577586341]
  Demux/8 -> [T79_6601_10018273794664]
  Demux/9 -> [T79_6602_10018864576563]
  Demux/10 -> [T79_6603_10019675735424]
  Demux/11 -> [T79_6602_10014889306339]
  Demux/12 -> [T79_6603_10015479073778]
  Demux/13 -> [T79_6604_10016289218179]
  Demux/14 -> [T56_4702_4750302846636]
  Demux/15 -> [T56_4703_4752532395919]
  Demux/16 -> [T56_4704_4754899674130]

== system SSN_39busRT_Ctrl_4WT_19B/powergui/EquivalentModel8/Sources ==
  Mux : Mux  Inputs=[2 1 1 1]
  u : Outport  VectorParamsAs1DForOutWhenUnconnected=off
  wires:
  Mux/1 -> u/1
  [T65_5755_7318402324279] -> Mux/1
  [T77_6302_8559278892273] -> Mux/2
  [T77_6303_8560525113701] -> Mux/3
  [T77_6304_8561997436169] -> Mux/4

== system SSN_39busRT_Ctrl_4WT_19B/powergui/EquivalentModel8/Yout ==
  v,i : Inport
  Demux : Demux  Outputs=[2 1 1 1 1 1 1 1 1 1 1 1 1]
  tag scope: T55_4659_4621905228909=global, T55_4660_4623978361515=global, T55_4661_4626185917394=global, T56_4731_4740040437805=global, T56_4732_4741880335192=global, T56_4733_4744290332724=global, T56_4737_4733971428179=global, T56_4738_4735800194429=global, T56_4739_4738198331221=global, T65_5750_7254415176404=global, T80_6660_10246361790872=global, T80_6661_10247019332720=global, T80_6662_10247900603568=global
  wires:
  v,i/1 -> Demux/1
  Demux/1 -> [T65_5750_7254415176404]
  Demux/2 -> [T56_4737_4733971428179]
  Demux/3 -> [T56_4739_4738198331221]
  Demux/4 -> [T56_4738_4735800194429]
  Demux/5 -> [T56_4731_4740040437805]
  Demux/6 -> [T56_4733_4744290332724]
  Demux/7 -> [T56_4732_4741880335192]
  Demux/8 -> [T80_6660_10246361790872]
  Demux/9 -> [T80_6661_10247019332720]
  Demux/10 -> [T80_6662_10247900603568]
  Demux/11 -> [T55_4659_4621905228909]
  Demux/12 -> [T55_4660_4623978361515]
  Demux/13 -> [T55_4661_4626185917394]

== system SSN_39busRT_Ctrl_4WT_19B/powergui/EquivalentModel9/Sources ==
  Mux : Mux  Inputs=[4 1 1 1 1 1 1 1]
  u : Outport  VectorParamsAs1DForOutWhenUnconnected=off
  wires:
  Mux/1 -> u/1
  [T174_15328_52553236377076] -> Mux/1
  [T159_13818_39553751375383] -> Mux/2
  [T159_13820_39606341578085] -> Mux/3
  [T160_13867_39435232525798] -> Mux/4
  [T160_13869_39488427681201] -> Mux/5
  [T75_6193_8152227292479] -> Mux/6
  [T75_6194_8153319948025] -> Mux/7
  [T75_6195_8154631976638] -> Mux/8

== system SSN_39busRT_Ctrl_4WT_19B/powergui/EquivalentModel9/Yout ==
  v,i : Inport
  Demux : Demux  Outputs=[4 1 1 1 1 1 1 1 1 1 1 1 1 1 1 1 1 1 1 1 1 1 1 1 1 1 1 1 1]
  tag scope: T123_10510_23699724775431=global, T123_10511_23706755090169=global, T123_10512_23714147366533=global, T123_10522_23834594266643=global, T123_10523_23841589599022=global, T123_10524_23848946893027=global, T159_13642_38339781814742=global, T159_13643_38349556408548=global, T159_13644_38359814222480=global, T159_13654_38527022724529=global, T159_13655_38536761104913=global, T159_13656_38546982705422=global, T165_14472_44791557802803=global, T165_14474_44839308485171=global, T166_14521_44775329845941=global, T166_14523_44823664606230=global, T174_15323_52379395362420=global, T175_15659_56226319845985=global, T176_15708_56043154866182=global, T176_15708_56375999222384=global, T176_15709_56043965003531=global, T176_15709_56373852619271=global, T177_15757_56194446161087=global, T177_15758_56192297040837=global, T177_15758_56195382605810=global, T177_15759_56193230745229=global, T78_6551_9768029206154=global, T78_6552_9768541673420=global, T78_6553_9769271166327=global
  wires:
  v,i/1 -> Demux/1
  Demux/1 -> [T174_15323_52379395362420]
  Demux/2 -> [T123_10522_23834594266643]
  Demux/3 -> [T123_10523_23841589599022]
  Demux/4 -> [T123_10524_23848946893027]
  Demux/5 -> [T159_13654_38527022724529]
  Demux/6 -> [T159_13655_38536761104913]
  Demux/7 -> [T159_13656_38546982705422]
  Demux/8 -> [T78_6551_9768029206154]
  Demux/9 -> [T78_6552_9768541673420]
  Demux/10 -> [T78_6553_9769271166327]
  Demux/11 -> [T123_10510_23699724775431]
  Demux/12 -> [T123_10511_23706755090169]
  Demux/13 -> [T123_10512_23714147366533]
  Demux/14 -> [T165_14472_44791557802803]
  Demux/15 -> [T165_14474_44839308485171]
  Demux/16 -> [T166_14521_44775329845941]
  Demux/17 -> [T166_14523_44823664606230]
  Demux/18 -> [T159_13642_38339781814742]
  Demux/19 -> [T159_13643_38349556408548]
  Demux/20 -> [T159_13644_38359814222480]
  Demux/21 -> [T175_15659_56226319845985]
  Demux/22 -> [T176_15708_56043154866182]
  Demux/23 -> [T176_15709_56043965003531]
  Demux/24 -> [T176_15708_56375999222384]
  Demux/25 -> [T177_15757_56194446161087]
  Demux/26 -> [T177_15758_56195382605810]
  Demux/27 -> [T176_15709_56373852619271]
  Demux/28 -> [T177_15758_56192297040837]
  Demux/29 -> [T177_15759_56193230745229]
